simulink model "LoadCell_Lab"  (R2025a)
settings: Solver=FixedStepAuto  StartTime=0.0  StopTime=inf  RelTol=1e-3  EnableMultiTasking=on
libraries: stm32f4xxblockslib x8, dspstat3 x1
settings Model: STM32="{\"AnalogInput\":[{\"ID\":\"test_poten:20\"},{\"ID\":\"test_poten:28\"},{\"ID\":\"ADC_reader:28\"},{\"ID\":\"ADC_reader:20\"},{\"ID\":\"ADC_reader:14\"},{\"ID\":\"ADC_reader:11\"},{\"ID\":\"ADC_reader:8\"},{\"ID\":\"ADC_reader:5\"},{\"ID\":\"ADC_reader:1\"},{\"ID\":\"ADC_reader_simulink:14\"},{\"ID\":\"ADC_reader_simulink:11\"},{\"ID\":\"ADC_reader_simulink:8\"},{\"ID\":\"ADC_reader_simulink:5\"},{\"ID\":\"ADC_reader_simulink:1\"},{\"ID\":\"ADC_reader_simulink:28\"}],\"DigitalPortRead\":{\"ID\":\"ADC_reader_simulink:47\"}}"  Creator=ioonz  LastModifiedBy=tawan
settings OptimizationCC: DefaultParameterBehavior=Inlined  EnhancedBackFolding=on  PassReuseOutputArgsAs=Individual arguments  ZeroExternalMemoryAtStartup=off  ZeroInternalMemoryAtStartup=off  MaxStackSize=512  OptimizeBlockOrder=speed  DifferentSizesBufferReuse=on  OptimizationCustomize=off  EfficientTunableParamExpr=on
settings DebuggingCC: ParameterTunabilityLossMsg=error
settings HardwareCC: ProdBitPerPointer=32.0  ProdBitPerSizeT=32.0  ProdBitPerPtrDiffT=32.0  ProdLargestAtomicInteger=Long  ProdLargestAtomicFloat=Double  ProdWordSize=32.0  ProdLongLongMode=on  ProdHWDeviceType=ARM Compatible->ARM Cortex-M
settings SFSimCC: MATLABDynamicMemAlloc=off
settings RTWCC: SystemTargetFile=ert.tlc  HardwareBoard=STM32G4xx Based  TemplateMakefile=ert_default_tmf  Toolchain=GNU Tools for ARM Embedded Processors  Description=Embedded Coder
settings CodeAppCC: ForceParamTrailComments=on  IgnoreCustomStorageClasses=off  OperatorAnnotations=on  SimulinkDataObjDesc=on  SFDataObjDesc=on  InsertBlockDesc=on
settings ERTTargetCC: ExtModeTransport=3.0  ExtModeStaticAllocSize=2048.0  TargetLangStandard=C99 (ISO)  CodeReplacementLibrary=ARM Cortex-M

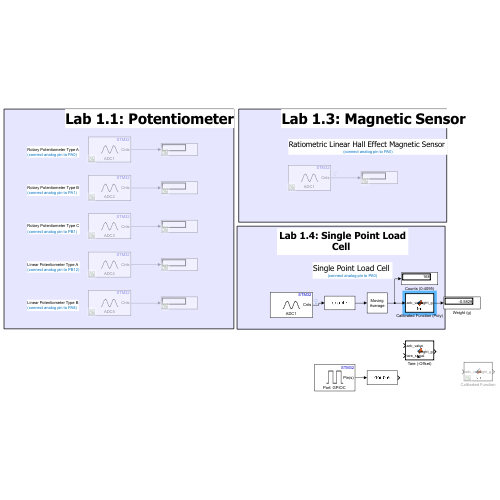
[thumbnail: Simulink's stored preview of the top-level diagram]
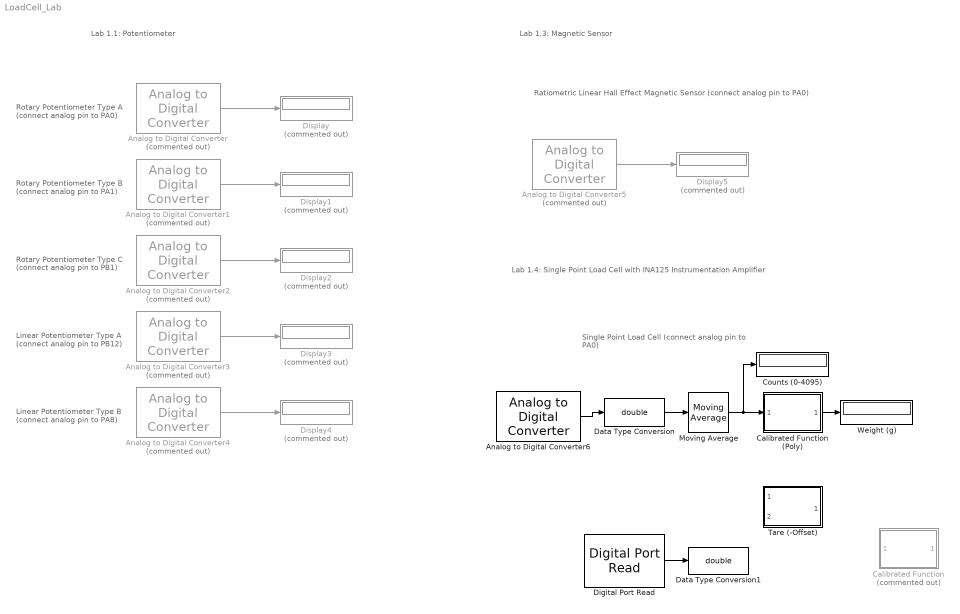
== system LoadCell_Lab ==
  note: Lab 1.1: Potentiometer
  note: Rotary Potentiometer Type A
      | (connect analog pin to PA0)
  note: Rotary Potentiometer Type B
      | (connect analog pin to PA1)
  note: Rotary Potentiometer Type C
      | (connect analog pin to PB1)
  note: Linear Potentiometer Type A
      | (connect analog pin to PB12)
  note: Linear Potentiometer Type B
      | (connect analog pin to PA8)
  note: Ratiometric Linear Hall Effect Magnetic Sensor
      | (connect analog pin to PA0)
  note: Single Point Load Cell
      | (connect analog pin to PA0)
  note: Lab 1.3: Magnetic Sensor
  note: Lab 1.4: Single Point Load Cell
      | with INA125 Instrumentation Amplifier
  Analog to Digital Converter : stm32f4xxblockslib/Analog to Digital Converter  Commented=on  ADCModule=ADC1  ConversionGroup=Regular  TriggerMode=Trigger and read  NumberOfConversions=1  EnableBufferConv=off  BufferLength=1  OutputStatus=off  SampleTime=-1  EnableSimPort=off  hoistedMaskSrc=ECSoC/ECSimCodegen/Analog to Digital Converter
  Analog to Digital Converter1 : stm32f4xxblockslib/Analog to Digital Converter  Commented=on  ADCModule=ADC2  ConversionGroup=Regular  TriggerMode=Trigger and read  NumberOfConversions=1  EnableBufferConv=off  BufferLength=1  OutputStatus=off  SampleTime=-1  EnableSimPort=off  hoistedMaskSrc=ECSoC/ECSimCodegen/Analog to Digital Converter
  Analog to Digital Converter2 : stm32f4xxblockslib/Analog to Digital Converter  Commented=on  ADCModule=ADC3  ConversionGroup=Regular  TriggerMode=Trigger and read  NumberOfConversions=1  EnableBufferConv=off  BufferLength=1  OutputStatus=off  SampleTime=-1  EnableSimPort=off  hoistedMaskSrc=ECSoC/ECSimCodegen/Analog to Digital Converter
  Analog to Digital Converter3 : stm32f4xxblockslib/Analog to Digital Converter  Commented=on  ADCModule=ADC4  ConversionGroup=Regular  TriggerMode=Trigger and read  NumberOfConversions=1  EnableBufferConv=off  BufferLength=1  OutputStatus=off  SampleTime=-1  EnableSimPort=off  hoistedMaskSrc=ECSoC/ECSimCodegen/Analog to Digital Converter
  Analog to Digital Converter4 : stm32f4xxblockslib/Analog to Digital Converter  Commented=on  ADCModule=ADC5  ConversionGroup=Regular  TriggerMode=Trigger and read  NumberOfConversions=1  EnableBufferConv=off  BufferLength=1  OutputStatus=off  SampleTime=-1  EnableSimPort=off  hoistedMaskSrc=ECSoC/ECSimCodegen/Analog to Digital Converter
  Analog to Digital Converter5 : stm32f4xxblockslib/Analog to Digital Converter  Commented=on  ADCModule=ADC1  ConversionGroup=Regular  TriggerMode=Trigger and read  NumberOfConversions=1  EnableBufferConv=off  BufferLength=1  OutputStatus=off  SampleTime=-1  EnableSimPort=off  hoistedMaskSrc=ECSoC/ECSimCodegen/Analog to Digital Converter
  Analog to Digital Converter6 : stm32f4xxblockslib/Analog to Digital Converter  ADCModule=ADC1  ConversionGroup=Regular  TriggerMode=Trigger and read  NumberOfConversions=1  EnableBufferConv=off  BufferLength=1  OutputStatus=off  SampleTime=-1  EnableSimPort=off  hoistedMaskSrc=ECSoC/ECSimCodegen/Analog to Digital Converter
  Calibrated Function : MATLAB Function  Commented=on  TreatAsAtomicUnit=on
  Calibrated Function (Poly) : MATLAB Function  TreatAsAtomicUnit=on
  Counts (0-4095) : Display
  Data Type Conversion : DataTypeConversion  OutDataTypeStr=double  SaturateOnIntegerOverflow=off  RndMeth=Floor
  Data Type Conversion1 : DataTypeConversion  OutDataTypeStr=double  SaturateOnIntegerOverflow=off  RndMeth=Floor
  Digital Port Read : stm32f4xxblockslib/Digital Port Read  PortName=GPIOC  PinNumber=[13]  ReadOperation=on  IOAsArray=on  SampleTime=0.001  EnableSimPort=off  hoistedMaskSrc=ECSoC/ECSimCodegen/Digital Port Read
  Display{,1..5} (6 alike) : Display  Commented=on
  Moving Average : dspstat3/Moving Average  Method=Sliding window  ForgettingFactorPort=off  SpecifyWindowLength=on  WindowLength=100  OverlapLength=99  AllowArbitraryInputLength=off  ForgettingFactor=0.99  SimulateUsing=Interpreted execution
  Tare (-Offset) : MATLAB Function  TreatAsAtomicUnit=on
  Weight (g) : Display
  wires:
  Analog to Digital Converter/1 -> Display/1
  Analog to Digital Converter1/1 -> Display1/1
  Analog to Digital Converter2/1 -> Display2/1
  Analog to Digital Converter3/1 -> Display3/1
  Analog to Digital Converter4/1 -> Display4/1
  Analog to Digital Converter5/1 -> Display5/1
  Analog to Digital Converter6/1 -> Data Type Conversion/1
  Moving Average/1 -> Calibrated Function (Poly)/1(adc_value), Counts (0-4095)/1
  Data Type Conversion/1 -> Moving Average/1
  Digital Port Read/1 -> Data Type Conversion1/1
  Calibrated Function (Poly)/1(weight_g) -> Weight (g)/1

== matlab function LoadCell_Lab/Calibrated Function ==
  data: adc_value input; weight_g output
function weight_g = fcn(adc_value)

% กำหนดค่า m และ c ที่ได้จากการ Calibration
m = 5.2990;
c = -218.2892;

% คำนวณน้ำหนัก
weight_g = (m * adc_value) + c;

% (Optional) ป้องกันค่าน้ำหนักติดลบ
if weight_g < 0
    weight_g = 0;
end

== matlab function LoadCell_Lab/Calibrated Function (Poly) ==
  data: adc_value input; weight_g output
function weight_g = fcn(adc_value)
%#codegen
% -------------------------------------------------------------------------
% ฟังก์ชันคำนวณน้ำหนักเวอร์ชันสมบูรณ์
% - ใช้สมการ Polynomial Degree 2 เพื่อความแม่นยำ
% - มีฟังก์ชัน Tare อัตโนมัติเมื่อสัญญาณเสถียร
% -------------------------------------------------------------------------

% --- ประกาศตัวแปร Persistent ---
persistent weight_offset;
persistent state;
persistent stable_counter;
persistent last_adc_value;

% --- สมการสอบเทียบใหม่ (Polynomial Degree 2) ---
% ---!!! ค่า a, b, c จากผลการทดลองของคุณ !!!---
a = -0.000652;
b =  6.523590;
c = -620.324675;

% --- Initialization (ทำงานแค่ครั้งแรกสุด) ---
if isempty(state)
    state = 0; % เริ่มต้นที่สถานะ "รอเสถียร"
    stable_counter = 0;
    last_adc_value = adc_value;
    weight_offset = 0; % กำหนดค่าเริ่มต้น
end

% --- กำหนดค่าเริ่มต้นให้ Output ก่อนเข้า Switch ---
weight_g = 0;

% --- State Machine Logic ---
switch state
    case 0 % สถานะ 0: รอให้สัญญาณ Input เสถียร
        if abs(adc_value - last_adc_value) < 0.5
            stable_counter = stable_counter + 1;
        else
            stable_counter = 0;
        end
        
        if stable_counter >= 200
            state = 1;
        end
        
    case 1 % สถานะ 1: ทำการ Tare (ทำงานแค่ครั้งเดียว)
        % คำนวณน้ำหนักดิบด้วยสมการพหุนาม
        raw_weight = (a * adc_value^2) + (b * adc_value) + c;
        % บันทึกค่าน้ำหนักนี้ไว้เป็น Offset
        weight_offset = raw_weight;
        state = 2; % เปลี่ยนไปสถานะ "ทำงานปกติ"

    case 2 % สถานะ 2: ทำงานปกติ
        % คำนวณน้ำหนักดิบด้วยสมการพหุนาม
        raw_weight = (a * adc_value^2) + (b * adc_value) + c;
        % หักลบด้วย Offset ที่บันทึกไว้
        weight_g = raw_weight - weight_offset;
end

% อัปเดตค่า ADC ล่าสุดเพื่อใช้ในรอบถัดไป
last_adc_value = adc_value;

% ป้องกันค่าน้ำหนักติดลบ (หลังจาก Tare แล้ว)
if weight_g < 0 && state == 2
    weight_g = 0;
end

end

== matlab function LoadCell_Lab/Tare (-Offset) ==
  data: adc_value input; weight_g output; tare_signal input
function weight_g = fcn(adc_value, tare_signal)
%#codegen

persistent weight_offset;
persistent last_tare_signal; 

m = 5.2990;
c = -218.2892;

if isempty(weight_offset)
    weight_offset = (m * adc_value) + c;
    % กำหนดชนิดข้อมูลให้เป็น double อย่างชัดเจน
    last_tare_signal = double(1); 
end

% --- Edge Detection Logic for Tare ---
% Input 'tare_signal' ตอนนี้เป็น double แล้ว (0.0 หรือ 1.0)
if (tare_signal == 0) && (last_tare_signal == 1)
    weight_offset = (m * adc_value) + c;
end

% อัปเดตสถานะปุ่มล่าสุด
last_tare_signal = tare_signal;

% --- คำนวณน้ำหนักสุทธิ ---
raw_weight = (m * adc_value) + c;
weight_g = raw_weight - weight_offset;

end
